simulink model "AccPed_DrvDemDes"  (R2016b)
settings: configuration reference "CodeGenConfigSet" (kept outside this file)
values from neighbouring files (symbols this model uses):
  AccPed_facCompTot_C = Calibration.Parameter    [init_AccPed_DrvDemDes.m]    (also in init_AccPed_DrvDemDes_SIL.m = Simulink.Parameter)
  ACCPED_OVRRUNRMP_SY = uint8(1)    [init_AccPed_DrvDemDes.m]    (also in init_AccPed_DrvDemDes_SIL.m)
  AccPed_rBrk50_CUR = Calibration.Parameter    [init_AccPed_DrvDemDes.m]    (also in init_AccPed_DrvDemDes_SIL.m = Simulink.Parameter)
  AccPed_rBrk50_CURX = Calibration.Parameter    [init_AccPed_DrvDemDes.m]    (also in init_AccPed_DrvDemDes_SIL.m = Simulink.Parameter)
  ACCPED_REVGEARMAP_SY = uint8(1)    [init_AccPed_DrvDemDes.m]    (also in init_AccPed_DrvDemDes_SIL.m)
  AccPed_rThresPrp_C = Calibration.Parameter    [init_AccPed_DrvDemDes.m]    (also in init_AccPed_DrvDemDes_SIL.m = Simulink.Parameter)
  AccPed_rZero_C = Calibration.Parameter    [init_AccPed_DrvDemDes.m]    (also in init_AccPed_DrvDemDes_SIL.m = Simulink.Parameter)
  AccPed_swtBrkPrio_C = Calibration.Parameter    [init_AccPed_DrvDemDes.m]    (also in init_AccPed_DrvDemDes_SIL.m = Simulink.Parameter)
  AccPed_trqDemThres_C = Calibration.Parameter    [init_AccPed_DrvDemDes.m]    (also in init_AccPed_DrvDemDes_SIL.m = Simulink.Parameter)
  AccPed_trqPrp_MAP = Calibration.Parameter    [init_AccPed_DrvDemDes.m]    (also in init_AccPed_DrvDemDes_SIL.m = Simulink.Parameter)
  AccPed_trqPrp_MAPX = Calibration.Parameter    [init_AccPed_DrvDemDes.m]    (also in init_AccPed_DrvDemDes_SIL.m = Simulink.Parameter)
  AccPed_trqPrp_MAPY = Calibration.Parameter    [init_AccPed_DrvDemDes.m]    (also in init_AccPed_DrvDemDes_SIL.m = Simulink.Parameter)
  FACT_ONE = int16(1)    [init_AccPed_DrvDemDes.m]    (also in init_AccPed_DrvDemDes_SIL.m)
  MoFDrDem_trqEng_MAP = Calibration.Parameter    [init_AccPed_DrvDemDes.m]    (also in init_AccPed_DrvDemDes_SIL.m = Simulink.Parameter)
  MoFDrDem_trqEng_MAPX = Calibration.Parameter    [init_AccPed_DrvDemDes.m]    (also in init_AccPed_DrvDemDes_SIL.m = Simulink.Parameter)
  MoFDrDem_trqEng_MAPY = Calibration.Parameter    [init_AccPed_DrvDemDes.m]    (also in init_AccPed_DrvDemDes_SIL.m = Simulink.Parameter)
  MoFDrDem_trqEngRev_MAP = Calibration.Parameter    [init_AccPed_DrvDemDes.m]    (also in init_AccPed_DrvDemDes_SIL.m = Simulink.Parameter)
  MoFDrDem_trqEngRev_MAPX = Calibration.Parameter    [init_AccPed_DrvDemDes.m]    (also in init_AccPed_DrvDemDes_SIL.m = Simulink.Parameter)
  MoFDrDem_trqEngRev_MAPY = Calibration.Parameter    [init_AccPed_DrvDemDes.m]    (also in init_AccPed_DrvDemDes_SIL.m = Simulink.Parameter)
  MSTSHFT_SY = uint8(0)    [init_AccPed_DrvDemDes.m]    (also in init_AccPed_DrvDemDes_SIL.m)
  SigTst_swtAccPed_C = Calibration.Parameter    [init_AccPed_DrvDemDes.m]    (also in init_AccPed_DrvDemDes_SIL.m = Simulink.Parameter)
  SigTst_trqAccPed_C = Calibration.Parameter    [init_AccPed_DrvDemDes.m]    (also in init_AccPed_DrvDemDes_SIL.m = Simulink.Parameter)
  TRQPRPHIGH_ZERO = int16(0)    [init_AccPed_DrvDemDes.m]    (also in init_AccPed_DrvDemDes_SIL.m)
undefined symbols (not defined in the file or in its folder): EBrk_stPreSelMode_conv, HPUn_etaPmp_MAPY, Switch_conv
libraries: simulink x21
settings Model: Creator=lenovo  LastModifiedBy=bianxuyin
settings ConfigSetRef: SourceLocation=Base Workspace

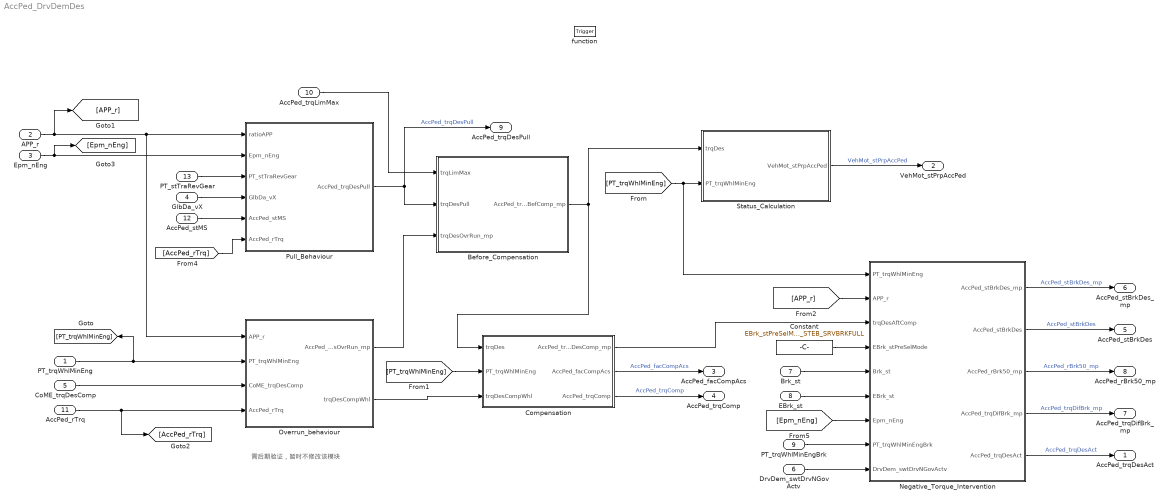
== system AccPed_DrvDemDes ==
  note: 需后期验证，暂时不修改该模块
  PT_trqWhlMinEng : Inport  Tag=Nm  Description=Minimum wheel torque from the engine  OutMin=-3000  OutMax=3000  OutDataTypeStr=Trq_Nm
  APP_r : Inport  Tag=%  Description=Acceleration pedal sensor 1 value after fault handling  Port=2  OutMin=0  OutMax=100  OutDataTypeStr=Accpedal_rate
  Epm_nEng : Inport  Tag=rpm  Description=Engine speed  Port=3  OutMin=0  OutMax=6000  OutDataTypeStr=EngSpeed_rpm
  GlbDa_vX : Inport  Tag=km/h  Description=Longitudinal vehicle speed (X-direction)  Port=4  OutMin=0  OutMax=250  OutDataTypeStr=VehSpeed_km_h
  CoME_trqDesComp : Inport  Tag=Nm  Description=Application parameter for torque demand of mechanical co-ordinator  Port=5  OutMin=-3000  OutMax=3000  OutDataTypeStr=Trq_Nm
  DrvDem_swtDrvNGovActv : Inport  Description=Switch to activate DrvDem  Port=6  OutDataTypeStr=Enum: Switch_conv
  Brk_st : Inport  Description=Brake switch state  Port=7  OutMin=0  OutMax=255  OutDataTypeStr=State_uint8
  EBrk_st : Inport  Description=Engine Brake switch status  Port=8  OutMin=0  OutMax=1  OutDataTypeStr=boolean
  PT_trqWhlMinEngBrk : Inport  Tag=Nm  Description=Minimum possible drag torque  Port=9  OutMin=-3000  OutMax=3000  OutDataTypeStr=Trq_Nm
  AccPed_trqLimMax : Inport  Tag=Nm  Description=Maximum wheel torque in case of accelerator pedal error  Port=10  OutMin=-3000  OutMax=3000  OutDataTypeStr=Trq_Nm
  AccPed_rTrq : Inport  Description=Total drive train ratio of engine - wheel  Port=11  OutMin=-327  OutMax=327  OutDataTypeStr=TransRatio
  AccPed_stMS : Inport  Description=Switch of the mastershift operation  Port=12  OutMin=0  OutMax=1  OutDataTypeStr=boolean
  PT_stTraRevGear : Inport  Description=Status if reverse gear is selected  Port=13  OutMin=0  OutMax=1  OutDataTypeStr=boolean
  function : TriggerPort  TriggerType=function-call  VariantControl=Variant
  Before_Compensation : Subsystem
  Compensation : Subsystem
  Constant : Constant  Value=EBrk_stPreSelMode_conv.EBPRESEL_STEB_SRVBRKFULL  OutDataTypeStr=Inherit: Inherit via back propagation
  Negative_Torque_Intervention : Subsystem
  Overrun_behaviour : Subsystem
  Pull_Behaviour : Subsystem
  Status_Calculation : Subsystem
  AccPed_trqDesAct : Outport  Tag=Nm  Description=driver torque raw of propulsion  OutMin=-3000  OutMax=3000  OutDataTypeStr=Trq_Nm
  VehMot_stPrpAccPed : Outport  Description=Status of propulsion demand by driver demand  Port=2  OutMin=0  OutMax=1  OutDataTypeStr=boolean
  AccPed_facCompAcs : Outport  Description="Factor \"Overrun Ramp\""  Port=3  OutMin=-4  OutMax=3.999  OutDataTypeStr=Fact8192
  AccPed_trqComp : Outport  Tag=Nm  Description=Compensation torque of accelerator pedal  Port=4  OutMin=-3000  OutMax=3000  OutDataTypeStr=Trq_Nm
  AccPed_stBrkDes : Outport  Description=Application parameter for engine brake request  Port=5  OutMin=0  OutMax=255  OutDataTypeStr=State_uint8
  AccPed_stBrkDes_mp : Outport  Description=raw engine brake request before prioritisation  Port=6  OutMin=0  OutMax=255  OutDataTypeStr=State_uint8
  AccPed_trqDifBrk_mp : Outport  Tag=Nm  Description=completely possible engine brake torque Nm  Port=7  OutMin=-3000  OutMax=3000  OutDataTypeStr=Trq_Nm
  AccPed_rBrk50_mp : Outport  Tag=%  Description=percentage of engine brake torque  Port=8  OutMin=0  OutMax=100  OutDataTypeStr=Accpedal_rate
  AccPed_trqDesPull : Outport  Tag=Nm  Description=Application parameter for driver demand in pull mode for desired value  Port=9  OutMin=-3000  OutMax=3000  OutDataTypeStr=Trq_Nm
  wires:
  Pull_Behaviour/1(AccPed_trqDesPull) -> AccPed_trqDesPull/1, Before_Compensation/2(trqDesPull)  "AccPed_trqDesPull"
  APP_r/1 -> Pull_Behaviour/1(ratioAPP), Overrun_behaviour/1(APP_r), [APP_r]
  PT_trqWhlMinEng/1 -> Overrun_behaviour/2(PT_trqWhlMinEng), [PT_trqWhlMinEng]
  CoME_trqDesComp/1 -> Overrun_behaviour/3(CoME_trqDesComp)
  AccPed_rTrq/1 -> Overrun_behaviour/4(AccPed_rTrq), [AccPed_rTrq]
  Compensation/1(AccPed_trqDesComp_mp) -> Negative_Torque_Intervention/3(trqDesAftComp)
  Status_Calculation/1(VehMot_stPrpAccPed) -> VehMot_stPrpAccPed/1  "VehMot_stPrpAccPed"
  AccPed_stMS/1 -> Pull_Behaviour/5(AccPed_stMS)
  GlbDa_vX/1 -> Pull_Behaviour/4(GlbDa_vX)
  [PT_trqWhlMinEng] -> Compensation/2("PT_trqWhlMinEng ")
  Compensation/2(AccPed_facCompAcs) -> AccPed_facCompAcs/1  "AccPed_facCompAcs"
  Compensation/3(AccPed_trqComp) -> AccPed_trqComp/1  "AccPed_trqComp"
  Negative_Torque_Intervention/1(AccPed_stBrkDes_mp) -> AccPed_stBrkDes_mp/1  "AccPed_stBrkDes_mp"
  Negative_Torque_Intervention/2(AccPed_stBrkDes) -> AccPed_stBrkDes/1  "AccPed_stBrkDes"
  [APP_r] -> Negative_Torque_Intervention/2(APP_r)
  Brk_st/1 -> Negative_Torque_Intervention/5(Brk_st)
  EBrk_st/1 -> Negative_Torque_Intervention/6(EBrk_st)
  [PT_trqWhlMinEng] -> Negative_Torque_Intervention/1(PT_trqWhlMinEng), Status_Calculation/2(PT_trqWhlMinEng)
  Epm_nEng/1 -> [Epm_nEng], Pull_Behaviour/2("Epm_nEng ")
  PT_trqWhlMinEngBrk/1 -> Negative_Torque_Intervention/8(PT_trqWhlMinEngBrk)
  Negative_Torque_Intervention/5(AccPed_trqDesAct) -> AccPed_trqDesAct/1  "AccPed_trqDesAct"
  Negative_Torque_Intervention/4(AccPed_trqDifBrk_mp) -> AccPed_trqDifBrk_mp/1  "AccPed_trqDifBrk_mp"
  Negative_Torque_Intervention/3(AccPed_rBrk50_mp) -> AccPed_rBrk50_mp/1  "AccPed_rBrk50_mp"
  DrvDem_swtDrvNGovActv/1 -> Negative_Torque_Intervention/9(DrvDem_swtDrvNGovActv)
  Before_Compensation/1(AccPed_trqDesBefComp_mp) -> Compensation/1(trqDes), Status_Calculation/1(trqDes)
  AccPed_trqLimMax/1 -> Before_Compensation/1(trqLimMax)
  Overrun_behaviour/1(AccPed_trqDesOvrRun_mp) -> Before_Compensation/3(trqDesOvrRun_mp)
  [AccPed_rTrq] -> Pull_Behaviour/6(AccPed_rTrq)
  [Epm_nEng] -> Negative_Torque_Intervention/7(Epm_nEng)
  Overrun_behaviour/2(trqDesCompWhl) -> Compensation/3(trqDesCompWhl)
  Constant/1 -> Negative_Torque_Intervention/4(EBrk_stPreSelMode)
  PT_stTraRevGear/1 -> Pull_Behaviour/3(PT_stTraRevGear)

== system AccPed_DrvDemDes/Before_Compensation ==
  trqLimMax : Inport
  trqDesPull : Inport  Port=2
  trqDesOvrRun_mp : Inport  Port=3
  Add : Sum  Inputs=+-  OutDataTypeStr=Inherit: Inherit via back propagation  SaturateOnIntegerOverflow=on  InputSameDT=on
  MinMax : MinMax  Inputs=2  InputSameDT=on
  AccPed_trqDesBefComp_mp : Outport
  wires:
  trqLimMax/1 -> MinMax/1
  Add/1 -> MinMax/2
  trqDesOvrRun_mp/1 -> Add/2
  MinMax/1 -> AccPed_trqDesBefComp_mp/1  "AccPed_trqDesBefComp_mp"
  trqDesPull/1 -> Add/1

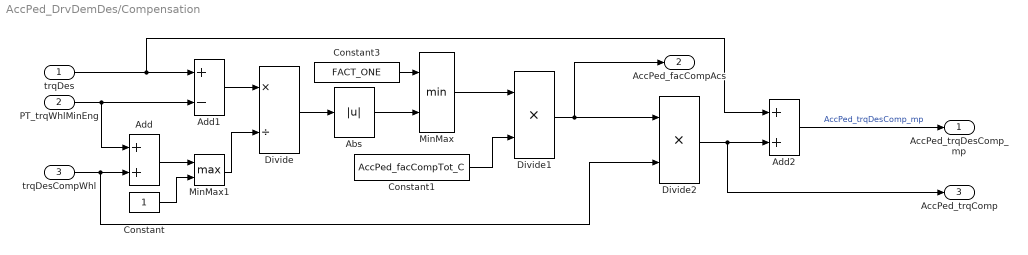
== system AccPed_DrvDemDes/Compensation ==
  trqDes : Inport
  "PT_trqWhlMinEng " : Inport  Port=2
  trqDesCompWhl : Inport  Port=3
  Abs : Abs
  Add : Sum  SaturateOnIntegerOverflow=on  InputSameDT=on
  Add1 : Sum  Inputs=+-  OutDataTypeStr=Inherit: Inherit via back propagation  SaturateOnIntegerOverflow=on  InputSameDT=on
  Add2 : Sum  SaturateOnIntegerOverflow=on  InputSameDT=on
  Constant : Constant  OutDataTypeStr=Inherit: Inherit via back propagation
  Constant1 : Constant  Value=AccPed_facCompTot_C
  Constant3 : Constant  Value=FACT_ONE  OutDataTypeStr=Factor
  Divide : Product  Inputs=*/  OutDataTypeStr=Factor  SaturateOnIntegerOverflow=on
  Divide1 : Product  Inputs=**  OutDataTypeStr=Inherit: Inherit via back propagation  SaturateOnIntegerOverflow=on
  Divide2 : Product  Inputs=**  OutDataTypeStr=Trq_Nm  SaturateOnIntegerOverflow=on
  MinMax : MinMax  Inputs=2  InputSameDT=on
  MinMax1 : MinMax  Function=max  Inputs=2
  AccPed_trqDesComp_mp : Outport  OutDataTypeStr=Trq_Nm
  AccPed_facCompAcs : Outport  Port=2
  AccPed_trqComp : Outport  Port=3
  wires:
  "PT_trqWhlMinEng "/1 -> Add1/2, Add/1
  trqDes/1 -> Add1/1, Add2/1
  Add1/1 -> Divide/1
  trqDesCompWhl/1 -> Add/2, Divide2/2
  Add/1 -> MinMax1/1
  Divide/1 -> Abs/1
  Abs/1 -> MinMax/2
  Constant3/1 -> MinMax/1
  MinMax/1 -> Divide1/1
  Constant1/1 -> Divide1/2
  Divide1/1 -> AccPed_facCompAcs/1, Divide2/1
  Divide2/1 -> AccPed_trqComp/1, Add2/2
  Add2/1 -> AccPed_trqDesComp_mp/1  "AccPed_trqDesComp_mp"
  MinMax1/1 -> Divide/2
  Constant/1 -> MinMax1/2

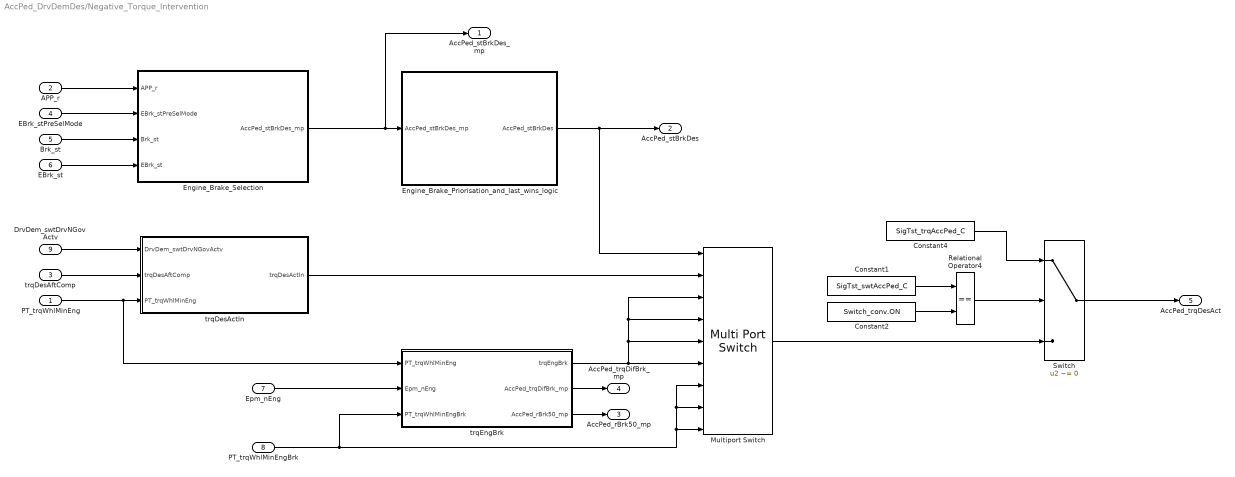
== system AccPed_DrvDemDes/Negative_Torque_Intervention ==
  PT_trqWhlMinEng : Inport
  APP_r : Inport  Port=2
  trqDesAftComp : Inport  Tag=-  Description=Switch to activate DrvDem  Port=3
  EBrk_stPreSelMode : Inport  Port=4
  Brk_st : Inport  Port=5
  EBrk_st : Inport  Port=6
  Epm_nEng : Inport  Port=7
  PT_trqWhlMinEngBrk : Inport  Port=8
  DrvDem_swtDrvNGovActv : Inport  Tag=-  Description=Switch to activate DrvDem  Port=9  OutDataTypeStr=Enum: Switch_conv
  Constant1 : Constant  Value=SigTst_swtAccPed_C
  Constant2 : Constant  Value=Switch_conv.ON  OutDataTypeStr=Inherit: Inherit via back propagation
  Constant4 : Constant  Value=SigTst_trqAccPed_C
  Engine_Brake_Priorisation_and_last_wins_logic : Subsystem
  Engine_Brake_Selection : Subsystem
  Multiport Switch : MultiPortSwitch  DataPortOrder=Specify indices  DataPortIndices={0,1,4,64,128,2,8,32}
  Relational Operator4 : RelationalOperator  Operator===  OutDataTypeStr=boolean  RndMeth=Simplest  InputSameDT=on
  Switch : Switch  Criteria=u2 ~= 0  InputSameDT=on
  trqDesActIn : Subsystem
  trqEngBrk : Subsystem
  AccPed_stBrkDes_mp : Outport
  AccPed_stBrkDes : Outport  Port=2
  AccPed_rBrk50_mp : Outport  Port=3
  AccPed_trqDifBrk_mp : Outport  Port=4
  AccPed_trqDesAct : Outport  Port=5
  wires:
  APP_r/1 -> Engine_Brake_Selection/1(APP_r)
  EBrk_stPreSelMode/1 -> Engine_Brake_Selection/2(EBrk_stPreSelMode)
  Brk_st/1 -> Engine_Brake_Selection/3(Brk_st)
  EBrk_st/1 -> Engine_Brake_Selection/4(EBrk_st)
  Engine_Brake_Selection/1(AccPed_stBrkDes_mp) -> AccPed_stBrkDes_mp/1, Engine_Brake_Priorisation_and_last_wins_logic/1(AccPed_stBrkDes_mp)
  Engine_Brake_Priorisation_and_last_wins_logic/1(AccPed_stBrkDes) -> Multiport Switch/1, AccPed_stBrkDes/1
  PT_trqWhlMinEngBrk/1 -> Multiport Switch/7, Multiport Switch/8, Multiport Switch/9, trqEngBrk/3(PT_trqWhlMinEngBrk)
  Multiport Switch/1 -> Switch/3
  Switch/1 -> AccPed_trqDesAct/1
  Constant4/1 -> Switch/1
  Constant1/1 -> Relational Operator4/1
  Constant2/1 -> Relational Operator4/2
  Relational Operator4/1 -> Switch/2
  PT_trqWhlMinEng/1 -> trqEngBrk/1(PT_trqWhlMinEng), trqDesActIn/3(PT_trqWhlMinEng)
  DrvDem_swtDrvNGovActv/1 -> trqDesActIn/1(DrvDem_swtDrvNGovActv)
  trqDesAftComp/1 -> trqDesActIn/2(trqDesAftComp)
  trqDesActIn/1(trqDesActIn) -> Multiport Switch/2
  trqEngBrk/1(trqEngBrk) -> Multiport Switch/3, Multiport Switch/4, Multiport Switch/5, Multiport Switch/6
  Epm_nEng/1 -> trqEngBrk/2(Epm_nEng)
  trqEngBrk/2(AccPed_trqDifBrk_mp) -> AccPed_trqDifBrk_mp/1
  trqEngBrk/3(AccPed_rBrk50_mp) -> AccPed_rBrk50_mp/1

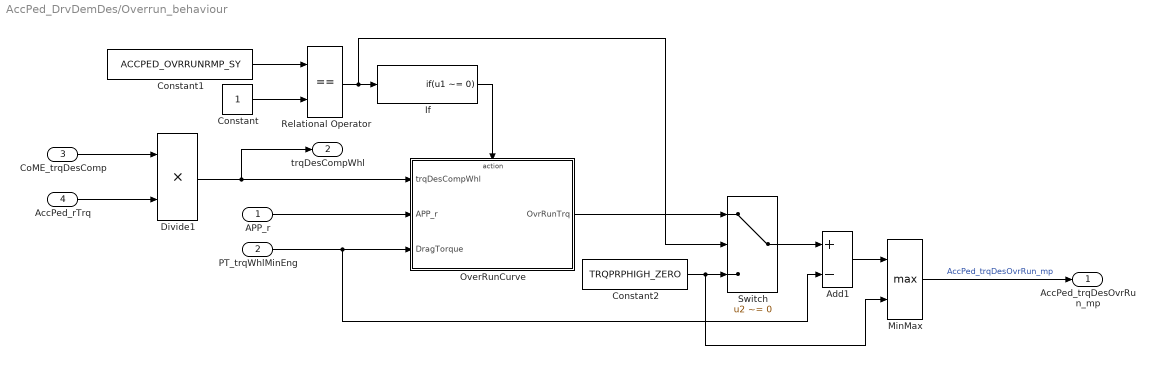
== system AccPed_DrvDemDes/Overrun_behaviour ==
  APP_r : Inport
  PT_trqWhlMinEng : Inport  Port=2
  CoME_trqDesComp : Inport  Tag=Nm  Description=Application parameter for torque demand of mechanical co-ordinator  Port=3  OutMin=-3000  OutMax=3000  OutDataTypeStr=Trq_Nm
  AccPed_rTrq : Inport  Tag=-  Description=Powertrain torque ratio  Port=4  OutMin=-327  OutMax=327  OutDataTypeStr=TransRatio
  Add1 : Sum  Inputs=+-  OutDataTypeStr=Inherit: Inherit via back propagation  SaturateOnIntegerOverflow=on  InputSameDT=on
  Constant : Constant  OutDataTypeStr=Inherit: Inherit via back propagation
  Constant1 : Constant  Value=ACCPED_OVRRUNRMP_SY
  Constant2 : Constant  Value=TRQPRPHIGH_ZERO  OutDataTypeStr=Trq_Nm
  Divide1 : Product  Inputs=**  OutDataTypeStr=Trq_Nm  SaturateOnIntegerOverflow=on
  If : If  IfExpression=u1 ~= 0  ShowElse=off
  MinMax : MinMax  Function=max  Inputs=2  InputSameDT=on
  OverRunCurve : Subsystem  TreatAsAtomicUnit=on
  Relational Operator : RelationalOperator  Operator===  OutDataTypeStr=boolean  RndMeth=Simplest  InputSameDT=on
  Switch : Switch  Criteria=u2 ~= 0  InputSameDT=on
  AccPed_trqDesOvrRun_mp : Outport
  trqDesCompWhl : Outport  Port=2
  wires:
  Constant1/1 -> Relational Operator/1
  Constant/1 -> Relational Operator/2
  Relational Operator/1 -> Switch/2, If/1
  If/1 -> OverRunCurve/Action
  OverRunCurve/1(OvrRunTrq) -> Switch/1
  Constant2/1 -> Switch/3, MinMax/2
  Switch/1 -> Add1/1
  Add1/1 -> MinMax/1
  MinMax/1 -> AccPed_trqDesOvrRun_mp/1  "AccPed_trqDesOvrRun_mp"
  APP_r/1 -> OverRunCurve/2(APP_r)
  Divide1/1 -> trqDesCompWhl/1, OverRunCurve/1(trqDesCompWhl)
  PT_trqWhlMinEng/1 -> Add1/2, OverRunCurve/3(DragTorque)
  CoME_trqDesComp/1 -> Divide1/1
  AccPed_rTrq/1 -> Divide1/2

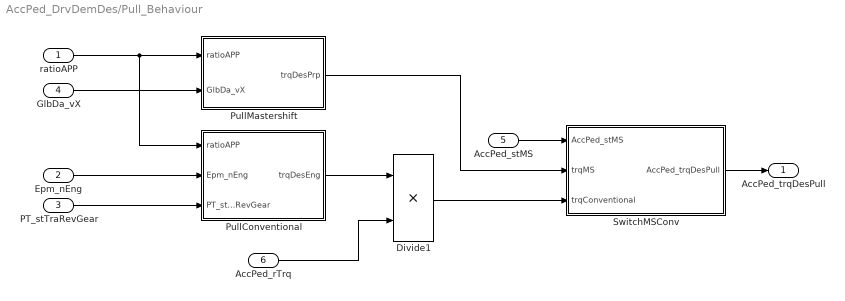
== system AccPed_DrvDemDes/Pull_Behaviour ==
  ratioAPP : Inport
  "Epm_nEng " : Inport  Port=2
  PT_stTraRevGear : Inport  Port=3
  GlbDa_vX : Inport  Port=4
  AccPed_stMS : Inport  Port=5
  AccPed_rTrq : Inport  Port=6
  Divide1 : Product  Inputs=**  OutDataTypeStr=Trq_Nm  SaturateOnIntegerOverflow=on
  PullConventional : Subsystem
  PullMastershift : Subsystem
  SwitchMSConv : Subsystem
  AccPed_trqDesPull : Outport
  wires:
  AccPed_rTrq/1 -> Divide1/2
  PullConventional/1(trqDesEng) -> Divide1/1
  Divide1/1 -> SwitchMSConv/3(trqConventional)
  PullMastershift/1(trqDesPrp) -> SwitchMSConv/2(trqMS)
  ratioAPP/1 -> PullConventional/1(ratioAPP), PullMastershift/1(ratioAPP)
  "Epm_nEng "/1 -> PullConventional/2("Epm_nEng ")
  PT_stTraRevGear/1 -> PullConventional/3(PT_stTraRevGear)
  GlbDa_vX/1 -> PullMastershift/2(GlbDa_vX)
  AccPed_stMS/1 -> SwitchMSConv/1(AccPed_stMS)
  SwitchMSConv/1(AccPed_trqDesPull) -> AccPed_trqDesPull/1

== system AccPed_DrvDemDes/Status_Calculation ==
  trqDes : Inport
  PT_trqWhlMinEng : Inport  Port=2
  Add : Sum  SaturateOnIntegerOverflow=on  InputSameDT=on
  Constant1 : Constant  Value=AccPed_trqDemThres_C
  Relational Operator : RelationalOperator  Operator=>  OutDataTypeStr=boolean  RndMeth=Simplest  InputSameDT=on
  VehMot_stPrpAccPed : Outport
  wires:
  trqDes/1 -> Relational Operator/1
  PT_trqWhlMinEng/1 -> Add/1
  Constant1/1 -> Add/2
  Add/1 -> Relational Operator/2
  Relational Operator/1 -> VehMot_stPrpAccPed/1

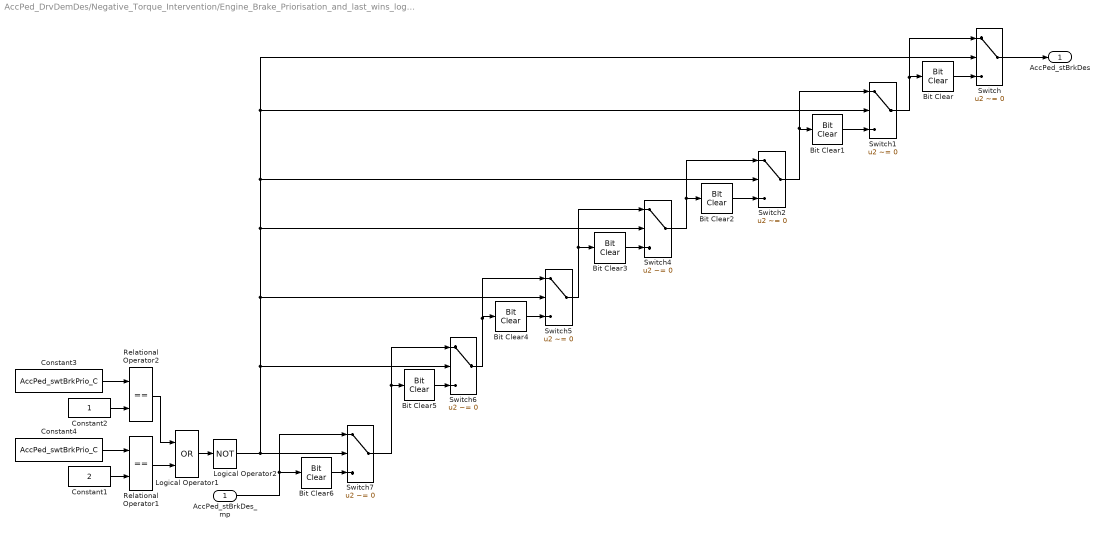
== system AccPed_DrvDemDes/Negative_Torque_Intervention/Engine_Brake_Priorisation_and_last_wins_logic ==
  AccPed_stBrkDes_mp : Inport
  Bit Clear : simulink/Logic and Bit Operations/Bit Clear  iBit=0
  Bit Clear1 : simulink/Logic and Bit Operations/Bit Clear  iBit=1
  Bit Clear2 : simulink/Logic and Bit Operations/Bit Clear  iBit=2
  Bit Clear3 : simulink/Logic and Bit Operations/Bit Clear  iBit=3
  Bit Clear4 : simulink/Logic and Bit Operations/Bit Clear  iBit=5
  Bit Clear5 : simulink/Logic and Bit Operations/Bit Clear  iBit=6
  Bit Clear6 : simulink/Logic and Bit Operations/Bit Clear  iBit=7
  Constant1 : Constant  Value=2  OutDataTypeStr=uint8
  Constant2 : Constant  OutDataTypeStr=uint8
  Constant3 : Constant  Value=AccPed_swtBrkPrio_C
  Constant4 : Constant  Value=AccPed_swtBrkPrio_C
  Logical Operator1 : Logic  Operator=OR  AllPortsSameDT=off  OutDataTypeStr=boolean
  Logical Operator2 : Logic  Operator=NOT  AllPortsSameDT=off  OutDataTypeStr=boolean
  Relational Operator1 : RelationalOperator  Operator===  OutDataTypeStr=boolean  RndMeth=Simplest
  Relational Operator2 : RelationalOperator  Operator===  OutDataTypeStr=boolean  RndMeth=Simplest
  Switch{,1..2,4..7} (7 alike) : Switch  Criteria=u2 ~= 0  InputSameDT=on
  AccPed_stBrkDes : Outport
  wires:
  Relational Operator1/1 -> Logical Operator1/2
  Logical Operator2/1 -> Switch7/2, Switch6/2, Switch5/2, Switch4/2, Switch2/2, Switch1/2, Switch/2
  Logical Operator1/1 -> Logical Operator2/1
  Bit Clear6/1 -> Switch7/3
  AccPed_stBrkDes_mp/1 -> Bit Clear6/1, Switch7/1
  Bit Clear5/1 -> Switch6/3
  Switch7/1 -> Bit Clear5/1, Switch6/1
  Bit Clear4/1 -> Switch5/3
  Switch6/1 -> Bit Clear4/1, Switch5/1
  Bit Clear3/1 -> Switch4/3
  Switch5/1 -> Bit Clear3/1, Switch4/1
  Bit Clear2/1 -> Switch2/3
  Switch4/1 -> Bit Clear2/1, Switch2/1
  Switch/1 -> AccPed_stBrkDes/1
  Bit Clear1/1 -> Switch1/3
  Switch2/1 -> Bit Clear1/1, Switch1/1
  Bit Clear/1 -> Switch/3
  Switch1/1 -> Bit Clear/1, Switch/1
  Relational Operator2/1 -> Logical Operator1/1
  Constant1/1 -> Relational Operator1/2
  Constant4/1 -> Relational Operator1/1
  Constant2/1 -> Relational Operator2/2
  Constant3/1 -> Relational Operator2/1

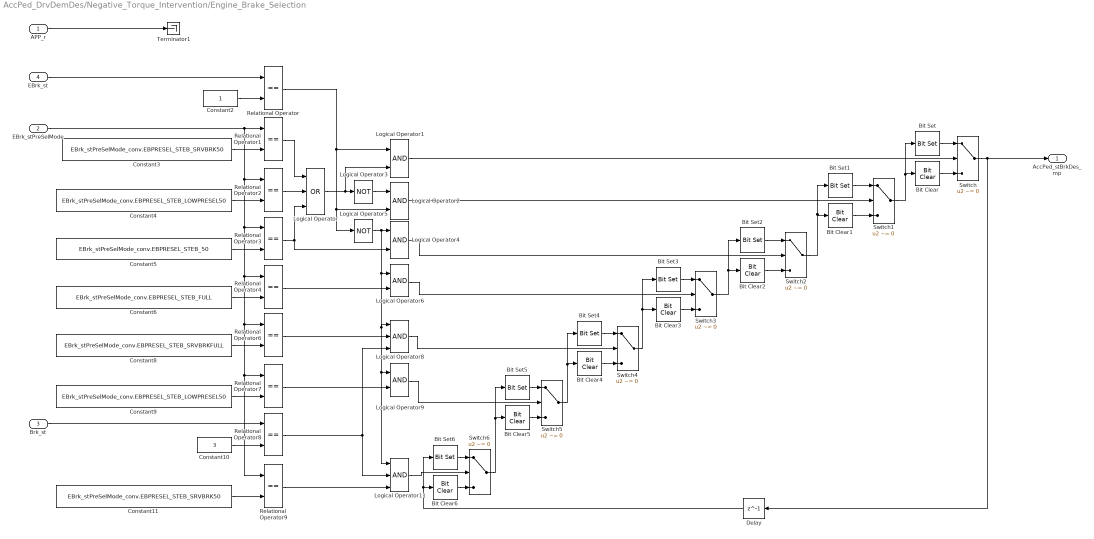
== system AccPed_DrvDemDes/Negative_Torque_Intervention/Engine_Brake_Selection ==
  APP_r : Inport
  EBrk_stPreSelMode : Inport  Port=2
  Brk_st : Inport  Port=3
  EBrk_st : Inport  Port=4
  Bit Clear : simulink/Logic and Bit Operations/Bit Clear  iBit=0
  Bit Clear1 : simulink/Logic and Bit Operations/Bit Clear  iBit=1
  Bit Clear2 : simulink/Logic and Bit Operations/Bit Clear  iBit=2
  Bit Clear3 : simulink/Logic and Bit Operations/Bit Clear  iBit=3
  Bit Clear4 : simulink/Logic and Bit Operations/Bit Clear  iBit=5
  Bit Clear5 : simulink/Logic and Bit Operations/Bit Clear  iBit=6
  Bit Clear6 : simulink/Logic and Bit Operations/Bit Clear  iBit=7
  Bit Set : simulink/Logic and Bit Operations/Bit Set  iBit=0
  Bit Set1 : simulink/Logic and Bit Operations/Bit Set  iBit=1
  Bit Set2 : simulink/Logic and Bit Operations/Bit Set  iBit=2
  Bit Set3 : simulink/Logic and Bit Operations/Bit Set  iBit=3
  Bit Set4 : simulink/Logic and Bit Operations/Bit Set  iBit=5
  Bit Set5 : simulink/Logic and Bit Operations/Bit Set  iBit=6
  Bit Set6 : simulink/Logic and Bit Operations/Bit Set  iBit=7
  Constant10 : Constant  Value=3  OutDataTypeStr=uint8
  Constant11 : Constant  Value=EBrk_stPreSelMode_conv.EBPRESEL_STEB_SRVBRK50
  Constant2 : Constant  OutDataTypeStr=uint8
  Constant3 : Constant  Value=EBrk_stPreSelMode_conv.EBPRESEL_STEB_SRVBRK50
  Constant4 : Constant  Value=EBrk_stPreSelMode_conv.EBPRESEL_STEB_LOWPRESEL50
  Constant5 : Constant  Value=EBrk_stPreSelMode_conv.EBPRESEL_STEB_50
  Constant6 : Constant  Value=EBrk_stPreSelMode_conv.EBPRESEL_STEB_FULL
  Constant8 : Constant  Value=EBrk_stPreSelMode_conv.EBPRESEL_STEB_SRVBRKFULL
  Constant9 : Constant  Value=EBrk_stPreSelMode_conv.EBPRESEL_STEB_LOWPRESEL50
  Delay : Delay  DelayLength=1  InitialCondition=0
  Logical Operator : Logic  Operator=OR  Inputs=3  AllPortsSameDT=off  OutDataTypeStr=boolean
  Logical Operator{1..2,4,6,9} (5 alike) : Logic  AllPortsSameDT=off  OutDataTypeStr=boolean
  Logical Operator11 : Logic  Inputs=3  AllPortsSameDT=off  OutDataTypeStr=boolean
  Logical Operator3 : Logic  Operator=NOT  AllPortsSameDT=off  OutDataTypeStr=boolean
  Logical Operator5 : Logic  Operator=NOT  AllPortsSameDT=off  OutDataTypeStr=boolean
  Logical Operator8 : Logic  Inputs=3  AllPortsSameDT=off  OutDataTypeStr=boolean
  Relational Operator{,1..4,6..9} (9 alike) : RelationalOperator  Operator===  OutDataTypeStr=boolean  RndMeth=Simplest
  Switch{,1..6} (7 alike) : Switch  Criteria=u2 ~= 0  InputSameDT=on
  Terminator1 : Terminator
  AccPed_stBrkDes_mp : Outport
  wires:
  Delay/1 -> Bit Clear6/1, Bit Set6/1
  Switch6/1 -> Bit Set5/1, Bit Clear5/1
  Logical Operator11/1 -> Switch6/2
  Bit Clear6/1 -> Switch6/3
  Bit Set6/1 -> Switch6/1
  Logical Operator9/1 -> Switch5/2
  Switch5/1 -> Bit Set4/1, Bit Clear4/1
  Bit Clear5/1 -> Switch5/3
  Bit Set5/1 -> Switch5/1
  Switch4/1 -> Bit Set3/1, Bit Clear3/1
  Logical Operator8/1 -> Switch4/2
  Bit Clear4/1 -> Switch4/3
  Bit Set4/1 -> Switch4/1
  Switch3/1 -> Bit Set2/1, Bit Clear2/1
  Logical Operator6/1 -> Switch3/2
  Bit Clear3/1 -> Switch3/3
  Bit Set3/1 -> Switch3/1
  Switch2/1 -> Bit Set1/1, Bit Clear1/1
  Logical Operator4/1 -> Switch2/2
  Bit Clear2/1 -> Switch2/3
  Bit Set2/1 -> Switch2/1
  Switch/1 -> Delay/1, AccPed_stBrkDes_mp/1
  Switch1/1 -> Bit Set/1, Bit Clear/1
  Logical Operator2/1 -> Switch1/2
  Bit Clear1/1 -> Switch1/3
  Bit Set1/1 -> Switch1/1
  Logical Operator1/1 -> Switch/2
  Bit Clear/1 -> Switch/3
  Bit Set/1 -> Switch/1
  Relational Operator9/1 -> Logical Operator11/3
  Relational Operator8/1 -> Logical Operator11/2, Logical Operator8/3
  Relational Operator7/1 -> Logical Operator9/2
  Constant11/1 -> Relational Operator9/2
  Constant10/1 -> Relational Operator8/2
  Constant9/1 -> Relational Operator7/2
  Relational Operator6/1 -> Logical Operator8/2
  Constant8/1 -> Relational Operator6/2
  Relational Operator4/1 -> Logical Operator6/2
  Logical Operator/1 -> Logical Operator1/2, Logical Operator3/1
  Relational Operator/1 -> Logical Operator5/1, Logical Operator2/2, Logical Operator1/1
  Logical Operator5/1 -> Logical Operator4/1, Logical Operator6/1, Logical Operator9/1, Logical Operator11/1, Logical Operator8/1
  Logical Operator3/1 -> Logical Operator2/1
  Relational Operator3/1 -> Logical Operator/3, Logical Operator4/2
  Relational Operator1/1 -> Logical Operator/1
  Relational Operator2/1 -> Logical Operator/2
  Constant6/1 -> Relational Operator4/2
  Constant5/1 -> Relational Operator3/2
  Constant4/1 -> Relational Operator2/2
  Constant3/1 -> Relational Operator1/2
  Constant2/1 -> Relational Operator/2
  APP_r/1 -> Terminator1/1
  EBrk_stPreSelMode/1 -> Relational Operator1/1, Relational Operator2/1, Relational Operator3/1, Relational Operator6/1, Relational Operator7/1, Relational Operator9/1, Relational Operator4/1
  Brk_st/1 -> Relational Operator8/1
  EBrk_st/1 -> Relational Operator/1

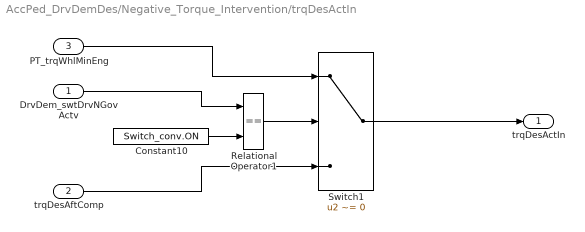
== system AccPed_DrvDemDes/Negative_Torque_Intervention/trqDesActIn ==
  DrvDem_swtDrvNGovActv : Inport  Tag=-  Description=Switch to activate DrvDem  OutDataTypeStr=Enum: Switch_conv
  trqDesAftComp : Inport  Tag=-  Description=Switch to activate DrvDem  Port=2
  PT_trqWhlMinEng : Inport  Port=3
  Constant10 : Constant  Value=Switch_conv.ON  OutDataTypeStr=Inherit: Inherit via back propagation
  Relational Operator1 : RelationalOperator  Operator===  OutDataTypeStr=boolean  RndMeth=Simplest  InputSameDT=on
  Switch1 : Switch  Criteria=u2 ~= 0  OutDataTypeStr=Inherit: Inherit via back propagation
  trqDesActIn : Outport
  wires:
  PT_trqWhlMinEng/1 -> Switch1/1
  Switch1/1 -> trqDesActIn/1
  trqDesAftComp/1 -> Switch1/3
  Constant10/1 -> Relational Operator1/2
  DrvDem_swtDrvNGovActv/1 -> Relational Operator1/1
  Relational Operator1/1 -> Switch1/2

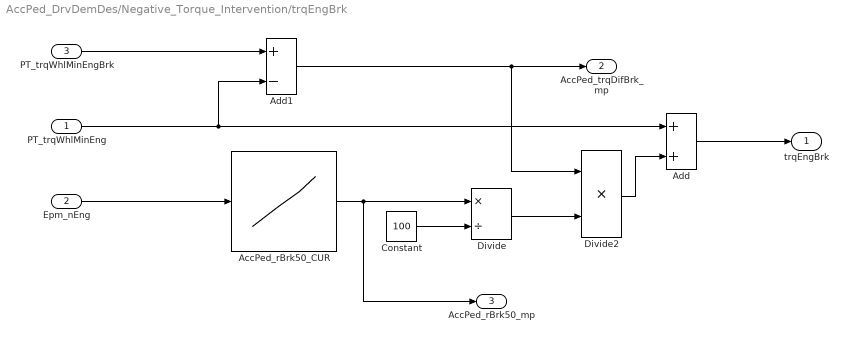
== system AccPed_DrvDemDes/Negative_Torque_Intervention/trqEngBrk ==
  PT_trqWhlMinEng : Inport
  Epm_nEng : Inport  Port=2
  PT_trqWhlMinEngBrk : Inport  Port=3
  AccPed_rBrk50_CUR : Lookup_n-D  NumberOfTableDimensions=1  BreakpointsForDimension1=AccPed_rBrk50_CURX  BreakpointsForDimension2=HPUn_etaPmp_MAPY  IndexSearchMethod=Linear search  BeginIndexSearchUsingPreviousIndexResult=on  Table=AccPed_rBrk50_CUR  ExtrapMethod=Clip  UseLastTableValue=on  InternalRulePriority=Speed  OutDataTypeStr=Inherit: Inherit via back propagation  SaturateOnIntegerOverflow=on
  Add : Sum  InputSameDT=on
  Add1 : Sum  Inputs=+-  OutDataTypeStr=Inherit: Inherit via back propagation  SaturateOnIntegerOverflow=on  InputSameDT=on
  Constant : Constant  Value=100  OutDataTypeStr=uint8
  Divide : Product  Inputs=*/  SaturateOnIntegerOverflow=on
  Divide2 : Product  Inputs=**  OutDataTypeStr=Trq_Nm  SaturateOnIntegerOverflow=on
  trqEngBrk : Outport
  AccPed_trqDifBrk_mp : Outport  Port=2
  AccPed_rBrk50_mp : Outport  Port=3
  wires:
  PT_trqWhlMinEngBrk/1 -> Add1/1
  PT_trqWhlMinEng/1 -> Add1/2, Add/1
  Epm_nEng/1 -> AccPed_rBrk50_CUR/1
  AccPed_rBrk50_CUR/1 -> Divide/1, AccPed_rBrk50_mp/1
  Add1/1 -> AccPed_trqDifBrk_mp/1, Divide2/1
  Divide2/1 -> Add/2
  Add/1 -> trqEngBrk/1
  Divide/1 -> Divide2/2
  Constant/1 -> Divide/2

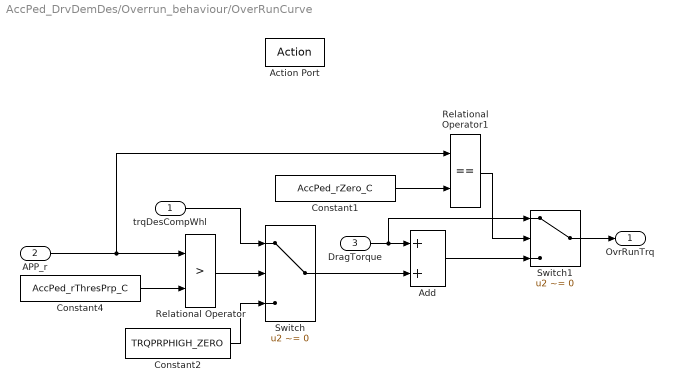
== system AccPed_DrvDemDes/Overrun_behaviour/OverRunCurve ==
  trqDesCompWhl : Inport
  APP_r : Inport  Port=2
  DragTorque : Inport  Port=3
  Action Port : ActionPort  ActionType=then
  Add : Sum  SaturateOnIntegerOverflow=on
  Constant1 : Constant  Value=AccPed_rZero_C  VectorParams1D=off
  Constant2 : Constant  Value=TRQPRPHIGH_ZERO  OutDataTypeStr=Trq_Nm
  Constant4 : Constant  Value=AccPed_rThresPrp_C
  Relational Operator : RelationalOperator  Operator=>  OutDataTypeStr=boolean  RndMeth=Simplest
  Relational Operator1 : RelationalOperator  Operator===  OutDataTypeStr=boolean  RndMeth=Simplest
  Switch : Switch  Criteria=u2 ~= 0  InputSameDT=on
  Switch1 : Switch  Criteria=u2 ~= 0  InputSameDT=on
  OvrRunTrq : Outport
  wires:
  DragTorque/1 -> Add/1, Switch1/1
  Switch1/1 -> OvrRunTrq/1
  Constant1/1 -> Relational Operator1/2
  Relational Operator1/1 -> Switch1/2
  Constant2/1 -> Switch/3
  Switch/1 -> Add/2
  Relational Operator/1 -> Switch/2
  APP_r/1 -> Relational Operator/1, Relational Operator1/1
  Constant4/1 -> Relational Operator/2
  trqDesCompWhl/1 -> Switch/1
  Add/1 -> Switch1/3

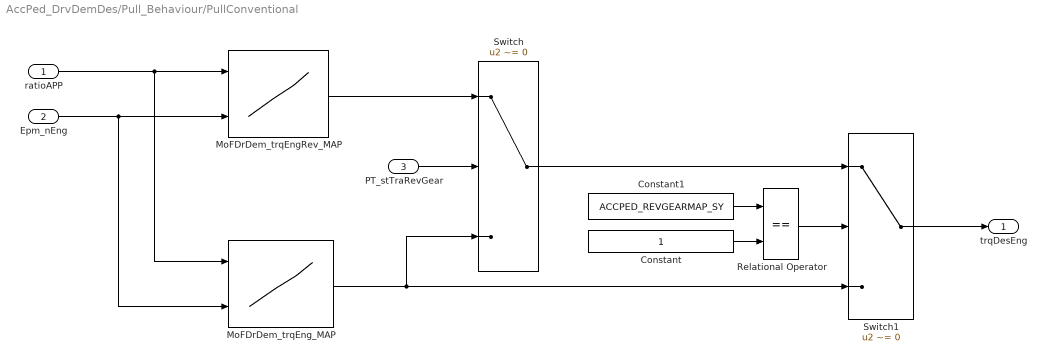
== system AccPed_DrvDemDes/Pull_Behaviour/PullConventional ==
  ratioAPP : Inport
  "Epm_nEng " : Inport  Port=2
  PT_stTraRevGear : Inport  Port=3
  Constant : Constant  OutDataTypeStr=Inherit: Inherit via back propagation
  Constant1 : Constant  Value=ACCPED_REVGEARMAP_SY
  MoFDrDem_trqEngRev_MAP : Lookup_n-D  BreakpointsForDimension1=MoFDrDem_trqEngRev_MAPY  BreakpointsForDimension2=MoFDrDem_trqEngRev_MAPX  IndexSearchMethod=Linear search  BeginIndexSearchUsingPreviousIndexResult=on  Table=MoFDrDem_trqEngRev_MAP  ExtrapMethod=Clip  UseLastTableValue=on  InternalRulePriority=Speed  OutDataTypeStr=Inherit: Inherit via back propagation  SaturateOnIntegerOverflow=on
  MoFDrDem_trqEng_MAP : Lookup_n-D  BreakpointsForDimension1=MoFDrDem_trqEng_MAPY  BreakpointsForDimension2=MoFDrDem_trqEng_MAPX  IndexSearchMethod=Linear search  BeginIndexSearchUsingPreviousIndexResult=on  Table=MoFDrDem_trqEng_MAP  ExtrapMethod=Clip  UseLastTableValue=on  InternalRulePriority=Speed  OutDataTypeStr=Inherit: Inherit via back propagation  SaturateOnIntegerOverflow=on
  Relational Operator : RelationalOperator  Operator===  OutDataTypeStr=boolean  RndMeth=Simplest  InputSameDT=on
  Switch : Switch  Criteria=u2 ~= 0  InputSameDT=on
  Switch1 : Switch  Criteria=u2 ~= 0  InputSameDT=on
  trqDesEng : Outport
  wires:
  Constant1/1 -> Relational Operator/1
  Constant/1 -> Relational Operator/2
  "Epm_nEng "/1 -> MoFDrDem_trqEng_MAP/2, MoFDrDem_trqEngRev_MAP/2
  ratioAPP/1 -> MoFDrDem_trqEng_MAP/1, MoFDrDem_trqEngRev_MAP/1
  MoFDrDem_trqEng_MAP/1 -> Switch1/3, Switch/3
  PT_stTraRevGear/1 -> Switch/2
  MoFDrDem_trqEngRev_MAP/1 -> Switch/1
  Switch/1 -> Switch1/1
  Relational Operator/1 -> Switch1/2
  Switch1/1 -> trqDesEng/1

== system AccPed_DrvDemDes/Pull_Behaviour/PullMastershift ==
  ratioAPP : Inport
  GlbDa_vX : Inport  Port=2
  AccPed_trqPrp_MAP : Lookup_n-D  BreakpointsForDimension1=AccPed_trqPrp_MAPY  BreakpointsForDimension2=AccPed_trqPrp_MAPX  IndexSearchMethod=Linear search  BeginIndexSearchUsingPreviousIndexResult=on  Table=AccPed_trqPrp_MAP  ExtrapMethod=Clip  UseLastTableValue=on  InternalRulePriority=Speed  OutDataTypeStr=Inherit: Inherit via back propagation  SaturateOnIntegerOverflow=on
  trqDesPrp : Outport
  wires:
  GlbDa_vX/1 -> AccPed_trqPrp_MAP/2
  ratioAPP/1 -> AccPed_trqPrp_MAP/1
  AccPed_trqPrp_MAP/1 -> trqDesPrp/1

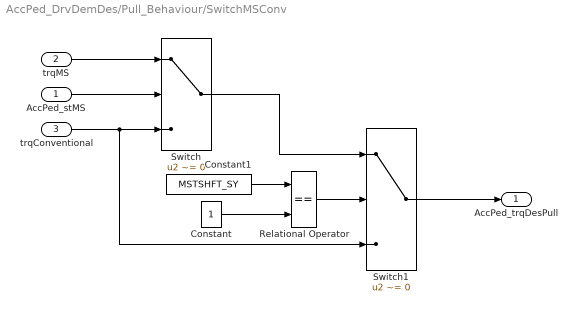
== system AccPed_DrvDemDes/Pull_Behaviour/SwitchMSConv ==
  AccPed_stMS : Inport
  trqMS : Inport  Port=2
  trqConventional : Inport  Port=3
  Constant : Constant  OutDataTypeStr=Inherit: Inherit via back propagation
  Constant1 : Constant  Value=MSTSHFT_SY
  Relational Operator : RelationalOperator  Operator===  OutDataTypeStr=boolean  RndMeth=Simplest  InputSameDT=on
  Switch : Switch  Criteria=u2 ~= 0  InputSameDT=on
  Switch1 : Switch  Criteria=u2 ~= 0  InputSameDT=on
  AccPed_trqDesPull : Outport
  wires:
  AccPed_stMS/1 -> Switch/2
  trqMS/1 -> Switch/1
  Relational Operator/1 -> Switch1/2
  Switch/1 -> Switch1/1
  trqConventional/1 -> Switch1/3, Switch/3
  Switch1/1 -> AccPed_trqDesPull/1
  Constant1/1 -> Relational Operator/1
  Constant/1 -> Relational Operator/2
